simulink model "fft_biplex_test3"  (Simulink 7.6)
settings: Solver=ode45  StartTime=0.0  StopTime=5000  RelTol=1e-3
libraries: xbsIndex_r4 x1382, casper_library x82, monroe_library x27, xps_library x17, dspsigops x16, simulink x1
(part 1 of 13)
settings Model: Creator=monroe  LastModifiedBy=monroe

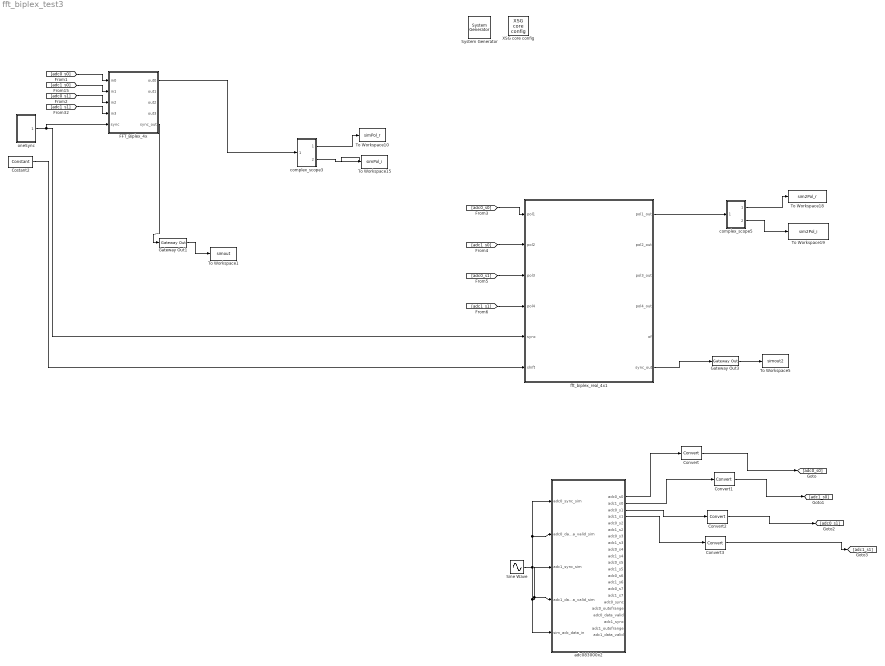
== system fft_biplex_test3 ==
  " System Generator" : xbsIndex_r4/ System Generator  Tag=genX  SystemSampleTime=-1  xilinxfamily=virtex5  part=xc5vsx95t  speed=-1  package=ff1136  synthesis_tool=XST  clock_wrapper=Clock Enables  directory=./spec_16in_extrabrams3/sysgen  testbench=off  simulink_period=1  sysclk_period=2.6667  dcm_input_clock_period=100  incr_netlist=off  trim_vbits=Everywhere in SubSystem  dbl_ovrd=According to Block Masks  core_generation=According to Block Masks  run_coregen=off  deprecated_control=off  eval_field=0  block_type=sysgen
      settings: block_version=11.4
  Convert{,1..3} (4 alike) : xbsIndex_r4/Convert  arith_type="Signed  (2's comp)"  n_bits=18  bin_pt=17  quantization=Truncate  overflow=Wrap  en=off  latency=0  dbl_ovrd=off  pipeline=off  block_type=convert
  Costant2 : xbsIndex_r4/Constant  arith_type=Signed (2's comp)  const=-1  n_bits=32  bin_pt=0  explicit_period=on  period=1  equ=P=C  opselect=C  inp2=PCIN>>17  opr=+  inp1=P  carry=CIN  dbl_ovrd=off  block_type=constant
      settings: block_version=11.4
  FFT_Biplex_4x : Subsystem  mask{FFTSize=10, coeff_bit_width=18*ones(1,8), input_bit_width=18, inter_stage_bit_width=18*ones(1,10), shift_arr=ones(1,10), max_distro_size_coeff=3, max_distro_size_delay=3, register_coeffs=0, stage_pre_delay=1, stage_mid_delay=1, stage_post_delay=0, bram_latency_fft=2, bram_latency_unscr=2, unscr_din_latency=0}
      mask prompts: FFTSize "FFT Size (2^?) points"; coeff_bit_width "Coefficient Bit Width"; input_bit_width "Input Bit Width"; inter_stage_bit_width "Inter-Stage Bit Widths"; shift_arr "Shift after n-th stage? (array of FFTSize elements, each a 0 or 1)"; max_distro_size_coeff "When to start putting Coefficients in BRAM (after 2^? elements)"; max_distro_size_delay "When to start putting Delays in BRAM (after 2^? latency)"; register_coeffs "Register Coefficients?"; stage_pre_delay "Stage Pre-delay? (0 or 1)"; stage_mid_delay "Stage Mid-Delay? (0 or 1)"; stage_post_delay "Stage Post-Delay? (0 or 1)"; bram_latency_fft "BRAM Latency (FFT)"; bram_latency_unscr "BRAM Latency (Unscrambler)"; unscr_din_latency "Unscrambler DIN Latency"
      mask init:
      | config.source=str2func('fft_biplex_4x_draw');
      | config.toplevel=gcb;
      | config.debug=0;
      | config.depend={'fft_biplex_4x_draw.m'};
      | xBlock(config,{FFTSize,coeff_bit_width,input_bit_width,inter_stage_bit_width,shift_arr,max_distro_size_coeff,max_distro_size_delay,register_coeffs,stage_pre_delay,stage_mid_delay,stage_post_delay,bram_latency_fft,bram_latency_unscr,unscr_din_latency});
  Gateway Out1 : xbsIndex_r4/Gateway Out  hdl_port=on  timing_constraint=None  locs_specified=off  LOCs={}  block_type=gatewayout
      settings: infoedit="Gateway out block.  Converts Xilinx fixed point inputs into ouputs of type Simulink integer, double, or fixed point.<br><br>Hardware notes:  In hardware these blocks become top level output ports or are discarded, depending on how they are configured."  block_version=11.4
  Gateway Out3 : xbsIndex_r4/Gateway Out  hdl_port=on  timing_constraint=None  locs_specified=off  LOCs={}  block_type=gatewayout
      settings: infoedit="Gateway out block.  Converts Xilinx fixed point inputs into ouputs of type Simulink integer, double, or fixed point.<br><br>Hardware notes:  In hardware these blocks become top level output ports or are discarded, depending on how they are configured."  block_version=11.4
  Sine Wave : Sin  Amplitude=.4  Frequency=1654.4/4096*pi*8  SampleTime=1/16
  To Workspace1 : ToWorkspace  VariableName=simout  SampleTime=-1  SaveFormat=Structure
  To Workspace10 : ToWorkspace  VariableName=simPol_r  SampleTime=-1  SaveFormat=Structure
  To Workspace15 : ToWorkspace  VariableName=simPol_i  SampleTime=-1  SaveFormat=Structure
  To Workspace18 : ToWorkspace  VariableName=sim2Pol_r  SampleTime=-1  SaveFormat=Structure
  To Workspace19 : ToWorkspace  VariableName=sim2Pol_i  SampleTime=-1  SaveFormat=Structure
  To Workspace5 : ToWorkspace  VariableName=simout2  SampleTime=-1  SaveFormat=Structure
  XSG core config : xps_library/XSG core config  Tag=xps:xsg  SystemSampleTime=-1  hw_sys=ROACH:sx95t  ibob_linux=off  clk_src=adc0_clk  iBOB_clk_src=sys_clk  BEE2_ctrl_clk_src=sys_clk  BEE2_usr_clk_src=sys_clk  ROACH_clk_src=adc0_clk  CORR_clk_src=sys_clk  gpio_clk_io_group=iBOB:sma  gpio_clk_bit_index=0  clk_rate=375  sample_period=1  synthesis_tool=XST  mpc_type=powerpc440_ext
  adc083000x2 : Subsystem  Tag=xps:adc083000x2  mask(adc_083000x2){use_adc0=on, use_adc1=on, demux_adc=off, clock_sync=off, verbose=on, using_ctrl=on, adc_clk_rate=1500, sample_period=1, bit_width=8}
      mask prompts: use_adc0 "Use ZD0K0?"; use_adc1 "Use ZDOK1?"; demux_adc "Demux ADCs by 2?"; clock_sync "Interleave 2 ADC boards?"; verbose "Verbose Block Creation?"; using_ctrl "Add ports for control registers?"; adc_clk_rate "ADC clock rate (MHz)"; sample_period "Sample Period"; bit_width "Output Bit Width"
      mask help:
      | The ADC block converts analog inputs to digital outputs.
      | Every clock cycle, the inputs are sampled and digitized to
      | 8 bit binary point numbers in the range of [-1, 1).
      |
      | Online block-specific documentation: http://casper.berkeley.edu/wiki/Adc083000
      mask Help: eval('xlWeb([getenv(''MLIB_ROOT''), ''\doc\html\sys_adc\sys_adc.html''])')
  complex_scope3 : Subsystem
  complex_scope5 : Subsystem
  fft_biplex_real_4x1 : Subsystem  AncestorBlock=casper_library/FFTs/fft_biplex_real_4x  mask(fft_biplex_real_4x){FFTSize=10, input_bit_width=8, coeff_bit_width=18, quantization=Truncate, overflow=Wrap, add_latency=2, mult_latency=3, bram_latency=3, arch=Virtex5, opt_target=Logic, coeffs_bit_limit=8, delays_bit_limit=9, specify_mult=off, mult_spec=, dsp48_adders=on, shifts=getfield( getfield( get_param( gcb,'UserData' ), 'parameters'),'shifts'), output_bit_widths=getfield( getfield( get_param( gcb,'UserData' ), 'parameters'),'output_bit_widths')}
      mask prompts: FFTSize "Size of FFT: (2^? pnts)"; input_bit_width "Input Bit Width"; coeff_bit_width "Coefficient Bit Width"; quantization "Quantization Behavior"; overflow "Overflow Behavior"; add_latency "Add Latency"; mult_latency "Mult Latency"; bram_latency "BRAM Latency"; arch "Architecture"; opt_target "Optimisation Target"; coeffs_bit_limit "Number bits above which to store stage's coefficients in BRAM (2^? bits)"; delays_bit_limit "Number bits above which to implement stage's delays in BRAM (2^? bits)"; specify_mult "Specify multiplier use (behavioral HDL if not specified)"; mult_spec "Multiplier specification (0=core, 1=embedded, 2=behavioural) (left=1st stage)"; dsp48_adders "Use DSP48s for adders"; shifts "Shift Schedule"; output_bit_widths "Output Bit Widths (vector len = nStages)"
      mask init:
      | fft_biplex_real_4x_init(gcb, ...
      |     'FFTSize', FFTSize, ...
      |     'input_bit_width', input_bit_width, ...
      |     'coeff_bit_width', coeff_bit_width, ...
      |     'quantization', quantization, ...
      |     'overflow', overflow, ...
      |     'add_latency', add_latency, ...
      |     'mult_latency', mult_latency, ...
      |     'bram_latency', bram_latency, ...
      |     'arch', arch, ...
      |     'opt_target', opt_target, ...
      |     'coeffs_bit_limit', coeffs_bit_limit, ...
      |     'delays_bit_limit', delays_bit_limit, ...    
      |     'specify_mult', specify_mult, ...
      |     'mult_spec', mult_spec, ...
      |     'dsp48_adders', dsp48_adders, ...
      |     'shifts', shifts, ...
      |     'output_bit_widths', output_bit_widths);
      settings: AttributesFormatString=FFTSize=10
      mask Help: eval('xlWeb(''http://casper.berkeley.edu/wiki/Fft_biplex_real_4x'')')
      mask StyleString: edit,edit,edit,popup(Truncate|Round  (unbiased: +/- Inf)|Round  (unbiased: Even Values)),popup(Wrap|Saturate|Error),edit,edit,edit,popup(Virtex2Pro|Virtex5),popup(Logic|Multipliers),edit,edit,checkbox,edit,checkbox,edit,edit
      mask CallbackString:
      | % fft_size = eval(get_param(gcb, 'FFTSize'));
      | % old_vec = eval(get_param(gcb, 'mult_spec'));
      | 
      | % vec = 2.*ones(1,fft_size);
      | % old_size = length(old_vec);
      | 
      | % if(old_size <= fft_size),
      | %     size = old_size;
      | % else,
      | %     size = fft_size;
      | % end
      | 
      | % for n = 1:size, vec(n) = old_vec(n); end
      | % set_param(gcb, 'mult_spec', mat2str(vec));||||||||||||specify_mult = get_param(gcb,'specify_mult');
      | visibs = get_param(gcb, 'MaskVisibilities');
      | enables = get_param(gcb, 'MaskEnables');
      | enables{14} = 'on';
      | if( strcmp(specify_mult,'off')), visibs{14} = 'off';
      | else, visibs{14} = 'on';
      | end
      | set_param(gcb, 'MaskVisibilities', visibs);
      | set_param(gcb, 'MaskEnables', enables);
      | |% vec = eval( get_param(gcb, 'mult_spec'));
      | % vec_size = length(vec);
      | % fft_size = eval( get_param(gcb, 'FFTSize'));
      | % new_vec = 2.*ones(1, fft_size);
      | 
      | % if(vec_size <= fft_size), size = vec_size;
      | % else size = fft_size;
      | % end
      | 
      | % for n=1:size
      | %    new_vec(n) = vec(n);
      | % end
      | % set_param(gcb, 'mult_spec', mat2str(new_vec));|||
  oneSync : Subsystem
  wires:
  [adc0_s0] -> FFT_Biplex_4x/1(in0)
  [adc1_s0] -> FFT_Biplex_4x/2(in1)
  [adc0_s1] -> FFT_Biplex_4x/3(in2)
  [adc1_s1] -> FFT_Biplex_4x/4(in3)
  oneSync/1(sync_out) -> fft_biplex_real_4x1/5(sync), FFT_Biplex_4x/5(sync)
  complex_scope3/1(Real) -> To Workspace10/1
  complex_scope3/2(Imag) -> To Workspace15/1
  FFT_Biplex_4x/5(sync_out) -> Gateway Out1/1
  Gateway Out1/1 -> To Workspace1/1
  [adc0_s0] -> fft_biplex_real_4x1/1(pol1)
  [adc1_s0] -> fft_biplex_real_4x1/2(pol2)
  [adc0_s1] -> fft_biplex_real_4x1/3(pol3)
  [adc1_s1] -> fft_biplex_real_4x1/4(pol4)
  complex_scope5/1(Real) -> To Workspace18/1
  complex_scope5/2(Imag) -> To Workspace19/1
  fft_biplex_real_4x1/1(pol1_out) -> complex_scope5/1(In1)
  Costant2/1 -> fft_biplex_real_4x1/6(shift)
  FFT_Biplex_4x/1(out0) -> complex_scope3/1(In1)
  Gateway Out3/1 -> To Workspace5/1
  fft_biplex_real_4x1/6(sync_out) -> Gateway Out3/1
  Sine Wave/1 -> adc083000x2/2(adc0_data_valid_sim), adc083000x2/1(adc0_sync_sim), adc083000x2/4(adc1_data_valid_sim), adc083000x2/3(adc1_sync_sim), adc083000x2/5(sim_adc_data_in)
  adc083000x2/1(adc0_s0) -> Convert/1
  adc083000x2/2(adc1_s0) -> Convert1/1
  adc083000x2/3(adc0_s1) -> Convert2/1
  adc083000x2/4(adc1_s1) -> Convert3/1
  Convert3/1 -> [adc1_s1]
  Convert2/1 -> [adc0_s1]
  Convert1/1 -> [adc1_s0]
  Convert/1 -> [adc0_s0]

== system fft_biplex_test3/FFT_Biplex_4x ==
  in0 : Inport
  in1 : Inport  Port=2
  in2 : Inport  Port=3
  in3 : Inport  Port=4
  sync : Inport  Port=5
  biplex_4x_unscr : Subsystem
  biplex_muxsel_gen : Subsystem
  coeff_slice10 : xbsIndex_r4/Slice  nbits=36  boolean_output=off  mode=Upper Bit Location + Width  bit1=-252  base1=MSB of Input  bit0=-252  base0=MSB of Input  dbl_ovrd=off  block_type=slice
  coeff_slice3 : xbsIndex_r4/Slice  nbits=36  boolean_output=off  mode=Upper Bit Location + Width  bit1=-0  base1=MSB of Input  bit0=-0  base0=MSB of Input  dbl_ovrd=off  block_type=slice
  coeff_slice4 : xbsIndex_r4/Slice  nbits=36  boolean_output=off  mode=Upper Bit Location + Width  bit1=-36  base1=MSB of Input  bit0=-36  base0=MSB of Input  dbl_ovrd=off  block_type=slice
  coeff_slice5 : xbsIndex_r4/Slice  nbits=36  boolean_output=off  mode=Upper Bit Location + Width  bit1=-72  base1=MSB of Input  bit0=-72  base0=MSB of Input  dbl_ovrd=off  block_type=slice
  coeff_slice6 : xbsIndex_r4/Slice  nbits=36  boolean_output=off  mode=Upper Bit Location + Width  bit1=-108  base1=MSB of Input  bit0=-108  base0=MSB of Input  dbl_ovrd=off  block_type=slice
  coeff_slice7 : xbsIndex_r4/Slice  nbits=36  boolean_output=off  mode=Upper Bit Location + Width  bit1=-144  base1=MSB of Input  bit0=-144  base0=MSB of Input  dbl_ovrd=off  block_type=slice
  coeff_slice8 : xbsIndex_r4/Slice  nbits=36  boolean_output=off  mode=Upper Bit Location + Width  bit1=-180  base1=MSB of Input  bit0=-180  base0=MSB of Input  dbl_ovrd=off  block_type=slice
  coeff_slice9 : xbsIndex_r4/Slice  nbits=36  boolean_output=off  mode=Upper Bit Location + Width  bit1=-216  base1=MSB of Input  bit0=-216  base0=MSB of Input  dbl_ovrd=off  block_type=slice
  cram0 : Subsystem
  cram1 : Subsystem
  sel_slice1 : xbsIndex_r4/Slice  nbits=1  boolean_output=on  mode=Upper Bit Location + Width  bit1=-0  base1=MSB of Input  bit0=-0  base0=MSB of Input  dbl_ovrd=off  block_type=slice
  sel_slice10 : xbsIndex_r4/Slice  nbits=1  boolean_output=on  mode=Upper Bit Location + Width  bit1=-9  base1=MSB of Input  bit0=-9  base0=MSB of Input  dbl_ovrd=off  block_type=slice
  sel_slice2 : xbsIndex_r4/Slice  nbits=1  boolean_output=on  mode=Upper Bit Location + Width  bit1=-1  base1=MSB of Input  bit0=-1  base0=MSB of Input  dbl_ovrd=off  block_type=slice
  sel_slice3 : xbsIndex_r4/Slice  nbits=1  boolean_output=on  mode=Upper Bit Location + Width  bit1=-2  base1=MSB of Input  bit0=-2  base0=MSB of Input  dbl_ovrd=off  block_type=slice
  sel_slice4 : xbsIndex_r4/Slice  nbits=1  boolean_output=on  mode=Upper Bit Location + Width  bit1=-3  base1=MSB of Input  bit0=-3  base0=MSB of Input  dbl_ovrd=off  block_type=slice
  sel_slice5 : xbsIndex_r4/Slice  nbits=1  boolean_output=on  mode=Upper Bit Location + Width  bit1=-4  base1=MSB of Input  bit0=-4  base0=MSB of Input  dbl_ovrd=off  block_type=slice
  sel_slice6 : xbsIndex_r4/Slice  nbits=1  boolean_output=on  mode=Upper Bit Location + Width  bit1=-5  base1=MSB of Input  bit0=-5  base0=MSB of Input  dbl_ovrd=off  block_type=slice
  sel_slice7 : xbsIndex_r4/Slice  nbits=1  boolean_output=on  mode=Upper Bit Location + Width  bit1=-6  base1=MSB of Input  bit0=-6  base0=MSB of Input  dbl_ovrd=off  block_type=slice
  sel_slice8 : xbsIndex_r4/Slice  nbits=1  boolean_output=on  mode=Upper Bit Location + Width  bit1=-7  base1=MSB of Input  bit0=-7  base0=MSB of Input  dbl_ovrd=off  block_type=slice
  sel_slice9 : xbsIndex_r4/Slice  nbits=1  boolean_output=on  mode=Upper Bit Location + Width  bit1=-8  base1=MSB of Input  bit0=-8  base0=MSB of Input  dbl_ovrd=off  block_type=slice
  stage_1 : Subsystem
  stage_10 : Subsystem
  stage_2 : Subsystem
  stage_3 : Subsystem
  stage_4 : Subsystem
  stage_5 : Subsystem
  stage_6 : Subsystem
  stage_7 : Subsystem
  stage_8 : Subsystem
  stage_9 : Subsystem
  out0 : Outport
  out1 : Outport  Port=2
  out2 : Outport  Port=3
  out3 : Outport  Port=4
  sync_out : Outport  Port=5
  wires:
  in0/1 -> cram0/1(in0)
  in1/1 -> cram0/2(in1)
  in2/1 -> cram1/1(in0)
  in3/1 -> cram1/2(in1)
  cram0/1(out) -> stage_1/1(a)
  cram1/1(out) -> stage_1/2(b)
  sel_slice1/1 -> stage_1/4(mux_sel)
  stage_1/1(a+bw) -> stage_2/1(a)
  stage_1/2(a-bw) -> stage_2/2(b)
  stage_1/3(sync_out) -> stage_2/3(sync)
  sel_slice2/1 -> stage_2/4(mux_sel)
  stage_2/1(a+bw) -> stage_3/1(a)
  stage_2/2(a-bw) -> stage_3/2(b)
  stage_2/3(sync_out) -> stage_3/3(sync)
  coeff_slice3/1 -> stage_3/4(coeff)
  sel_slice3/1 -> stage_3/5(mux_sel)
  stage_3/1(a+bw) -> stage_4/1(a)
  stage_3/2(a-bw) -> stage_4/2(b)
  stage_3/3(sync_out) -> stage_4/3(sync)
  coeff_slice4/1 -> stage_4/4(coeff)
  sel_slice4/1 -> stage_4/5(mux_sel)
  stage_4/1(a+bw) -> stage_5/1(a)
  stage_4/2(a-bw) -> stage_5/2(b)
  stage_4/3(sync_out) -> stage_5/3(sync)
  coeff_slice5/1 -> stage_5/4(coeff)
  sel_slice5/1 -> stage_5/5(mux_sel)
  stage_5/1(a+bw) -> stage_6/1(a)
  stage_5/2(a-bw) -> stage_6/2(b)
  stage_5/3(sync_out) -> stage_6/3(sync)
  coeff_slice6/1 -> stage_6/4(coeff)
  sel_slice6/1 -> stage_6/5(mux_sel)
  stage_6/1(a+bw) -> stage_7/1(a)
  stage_6/2(a-bw) -> stage_7/2(b)
  stage_6/3(sync_out) -> stage_7/3(sync)
  coeff_slice7/1 -> stage_7/4(coeff)
  sel_slice7/1 -> stage_7/5(mux_sel)
  stage_7/1(a+bw) -> stage_8/1(a)
  stage_7/2(a-bw) -> stage_8/2(b)
  stage_7/3(sync_out) -> stage_8/3(sync)
  coeff_slice8/1 -> stage_8/4(coeff)
  sel_slice8/1 -> stage_8/5(mux_sel)
  stage_8/1(a+bw) -> stage_9/1(a)
  stage_8/2(a-bw) -> stage_9/2(b)
  stage_8/3(sync_out) -> stage_9/3(sync)
  coeff_slice9/1 -> stage_9/4(coeff)
  sel_slice9/1 -> stage_9/5(mux_sel)
  stage_9/1(a+bw) -> stage_10/1(a)
  stage_9/2(a-bw) -> stage_10/2(b)
  stage_9/3(sync_out) -> stage_10/3(sync)
  coeff_slice10/1 -> stage_10/4(coeff)
  sel_slice10/1 -> stage_10/5(mux_sel)
  stage_10/1(a+bw) -> biplex_4x_unscr/1(even)
  stage_10/2(a-bw) -> biplex_4x_unscr/2(odd)
  biplex_muxsel_gen/3(sync_out) -> biplex_4x_unscr/3(sync)
  biplex_4x_unscr/1(pol1_out) -> out0/1
  biplex_4x_unscr/2(pol2_out) -> out1/1
  biplex_4x_unscr/3(pol3_out) -> out2/1
  biplex_4x_unscr/4(pol4_out) -> out3/1
  biplex_4x_unscr/5(sync_out) -> sync_out/1
  biplex_muxsel_gen/1(coeff) -> coeff_slice3/1, coeff_slice4/1, coeff_slice5/1, coeff_slice6/1, coeff_slice7/1, coeff_slice8/1, coeff_slice9/1, coeff_slice10/1
  biplex_muxsel_gen/2(sel) -> sel_slice1/1, sel_slice2/1, sel_slice3/1, sel_slice4/1, sel_slice5/1, sel_slice6/1, sel_slice7/1, sel_slice8/1, sel_slice9/1, sel_slice10/1
  sync/1 -> biplex_muxsel_gen/1(sync), stage_1/3(sync)

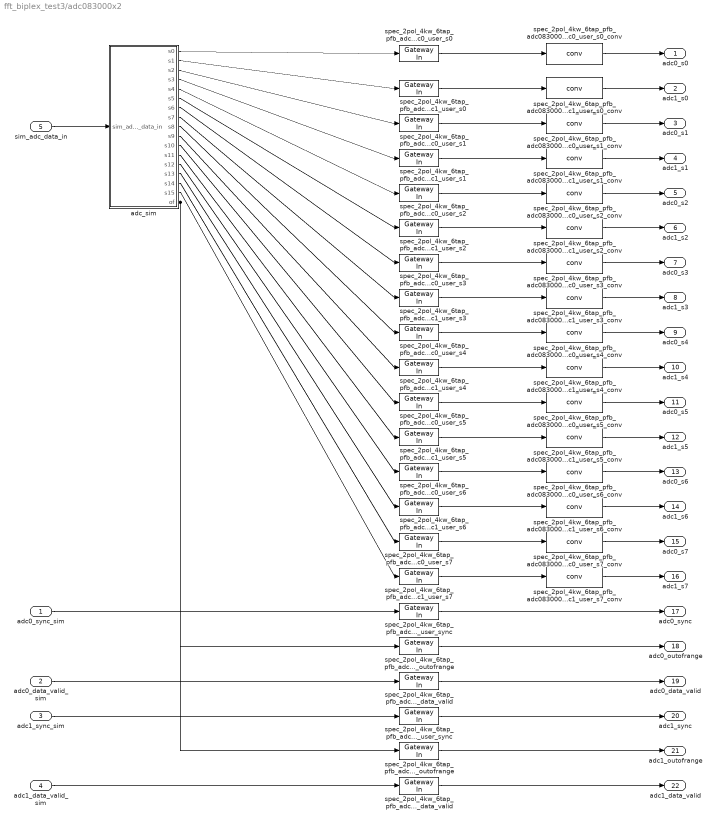
== system fft_biplex_test3/adc083000x2 ==
  adc0_sync_sim : Inport
  adc0_data_valid_sim : Inport  Port=2
  adc1_sync_sim : Inport  Port=3
  adc1_data_valid_sim : Inport  Port=4
  sim_adc_data_in : Inport  Port=5
  adc_sim : Subsystem  AncestorBlock=xps_library/ADCs/adc_sim  mask(adc_sim){nStreams=16, bit_width=8}
      mask prompts: nStreams "Number of Output Streams"; bit_width "Sample Bit Width"
      mask help:
      | This block simulates the behavior of a demuxed ADC, which takes
      | as input a waveform and returns digital samples in parallel at
      | a slower rate.
      |
      | This block is used to simulate the behavior
      mask init:
      | adc_sim_init(gcb, ...
      |     'nStreams', nStreams, ...
      |     'bit_width', bit_width);
  spec_2pol_4kw_6tap_pfb_adc083000x2_adc0_user_data_valid : xbsIndex_r4/Gateway In  arith_type=Unsigned  n_bits=1  bin_pt=0  quantization="Round  (unbiased: +/- Inf)"  overflow=Saturate  period=1  dbl_ovrd=off  timing_constraint=None  locs_specified=off  LOCs={}  hdl_port=on  block_type=gatewayin
      settings: infoedit="Gateway in block.  Converts inputs of type Simulink integer, double and fixed point to  Xilinx fixed point type.<br><br>Hardware notes:  In hardware these blocks become top level input ports."
  spec_2pol_4kw_6tap_pfb_adc083000x2_adc0_user_outofrange : xbsIndex_r4/Gateway In  arith_type=Unsigned  n_bits=4  bin_pt=0  quantization="Round  (unbiased: +/- Inf)"  overflow=Saturate  period=1  dbl_ovrd=off  timing_constraint=None  locs_specified=off  LOCs={}  hdl_port=on  block_type=gatewayin
      settings: infoedit="Gateway in block.  Converts inputs of type Simulink integer, double and fixed point to  Xilinx fixed point type.<br><br>Hardware notes:  In hardware these blocks become top level input ports."
  spec_2pol_4kw_6tap_pfb_adc083000x2_adc0_user_s{0..7} (8 alike) : xbsIndex_r4/Gateway In  arith_type=Unsigned  n_bits=8  bin_pt=0  quantization="Round  (unbiased: +/- Inf)"  overflow=Saturate  period=1  dbl_ovrd=off  timing_constraint=None  locs_specified=off  LOCs={}  hdl_port=on  block_type=gatewayin
      settings: infoedit="Gateway in block.  Converts inputs of type Simulink integer, double and fixed point to  Xilinx fixed point type.<br><br>Hardware notes:  In hardware these blocks become top level input ports."
  spec_2pol_4kw_6tap_pfb_adc083000x2_adc0_user_s0_conv : xps_library/ADCs/conv  SystemSampleTime=-1  bit_width=8
  spec_2pol_4kw_6tap_pfb_adc083000x2_adc0_user_s1_conv : xps_library/ADCs/conv  SystemSampleTime=-1  bit_width=8
  spec_2pol_4kw_6tap_pfb_adc083000x2_adc0_user_s2_conv : xps_library/ADCs/conv  SystemSampleTime=-1  bit_width=8
  spec_2pol_4kw_6tap_pfb_adc083000x2_adc0_user_s3_conv : xps_library/ADCs/conv  SystemSampleTime=-1  bit_width=8
  spec_2pol_4kw_6tap_pfb_adc083000x2_adc0_user_s4_conv : xps_library/ADCs/conv  SystemSampleTime=-1  bit_width=8
  spec_2pol_4kw_6tap_pfb_adc083000x2_adc0_user_s5_conv : xps_library/ADCs/conv  SystemSampleTime=-1  bit_width=8
  spec_2pol_4kw_6tap_pfb_adc083000x2_adc0_user_s6_conv : xps_library/ADCs/conv  SystemSampleTime=-1  bit_width=8
  spec_2pol_4kw_6tap_pfb_adc083000x2_adc0_user_s7_conv : xps_library/ADCs/conv  SystemSampleTime=-1  bit_width=8
  spec_2pol_4kw_6tap_pfb_adc083000x2_adc0_user_sync : xbsIndex_r4/Gateway In  arith_type=Unsigned  n_bits=4  bin_pt=0  quantization="Round  (unbiased: +/- Inf)"  overflow=Saturate  period=1  dbl_ovrd=off  timing_constraint=None  locs_specified=off  LOCs={}  hdl_port=on  block_type=gatewayin
      settings: infoedit="Gateway in block.  Converts inputs of type Simulink integer, double and fixed point to  Xilinx fixed point type.<br><br>Hardware notes:  In hardware these blocks become top level input ports."
  spec_2pol_4kw_6tap_pfb_adc083000x2_adc1_user_data_valid : xbsIndex_r4/Gateway In  arith_type=Unsigned  n_bits=1  bin_pt=0  quantization="Round  (unbiased: +/- Inf)"  overflow=Saturate  period=1  dbl_ovrd=off  timing_constraint=None  locs_specified=off  LOCs={}  hdl_port=on  block_type=gatewayin
      settings: infoedit="Gateway in block.  Converts inputs of type Simulink integer, double and fixed point to  Xilinx fixed point type.<br><br>Hardware notes:  In hardware these blocks become top level input ports."
  spec_2pol_4kw_6tap_pfb_adc083000x2_adc1_user_outofrange : xbsIndex_r4/Gateway In  arith_type=Unsigned  n_bits=4  bin_pt=0  quantization="Round  (unbiased: +/- Inf)"  overflow=Saturate  period=1  dbl_ovrd=off  timing_constraint=None  locs_specified=off  LOCs={}  hdl_port=on  block_type=gatewayin
      settings: infoedit="Gateway in block.  Converts inputs of type Simulink integer, double and fixed point to  Xilinx fixed point type.<br><br>Hardware notes:  In hardware these blocks become top level input ports."
  spec_2pol_4kw_6tap_pfb_adc083000x2_adc1_user_s{0..7} (8 alike) : xbsIndex_r4/Gateway In  arith_type=Unsigned  n_bits=8  bin_pt=0  quantization="Round  (unbiased: +/- Inf)"  overflow=Saturate  period=1  dbl_ovrd=off  timing_constraint=None  locs_specified=off  LOCs={}  hdl_port=on  block_type=gatewayin
      settings: infoedit="Gateway in block.  Converts inputs of type Simulink integer, double and fixed point to  Xilinx fixed point type.<br><br>Hardware notes:  In hardware these blocks become top level input ports."
  spec_2pol_4kw_6tap_pfb_adc083000x2_adc1_user_s0_conv : xps_library/ADCs/conv  SystemSampleTime=-1  bit_width=8
  spec_2pol_4kw_6tap_pfb_adc083000x2_adc1_user_s1_conv : xps_library/ADCs/conv  SystemSampleTime=-1  bit_width=8
  spec_2pol_4kw_6tap_pfb_adc083000x2_adc1_user_s2_conv : xps_library/ADCs/conv  SystemSampleTime=-1  bit_width=8
  spec_2pol_4kw_6tap_pfb_adc083000x2_adc1_user_s3_conv : xps_library/ADCs/conv  SystemSampleTime=-1  bit_width=8
  spec_2pol_4kw_6tap_pfb_adc083000x2_adc1_user_s4_conv : xps_library/ADCs/conv  SystemSampleTime=-1  bit_width=8
  spec_2pol_4kw_6tap_pfb_adc083000x2_adc1_user_s5_conv : xps_library/ADCs/conv  SystemSampleTime=-1  bit_width=8
  spec_2pol_4kw_6tap_pfb_adc083000x2_adc1_user_s6_conv : xps_library/ADCs/conv  SystemSampleTime=-1  bit_width=8
  spec_2pol_4kw_6tap_pfb_adc083000x2_adc1_user_s7_conv : xps_library/ADCs/conv  SystemSampleTime=-1  bit_width=8
  spec_2pol_4kw_6tap_pfb_adc083000x2_adc1_user_sync : xbsIndex_r4/Gateway In  arith_type=Unsigned  n_bits=4  bin_pt=0  quantization="Round  (unbiased: +/- Inf)"  overflow=Saturate  period=1  dbl_ovrd=off  timing_constraint=None  locs_specified=off  LOCs={}  hdl_port=on  block_type=gatewayin
      settings: infoedit="Gateway in block.  Converts inputs of type Simulink integer, double and fixed point to  Xilinx fixed point type.<br><br>Hardware notes:  In hardware these blocks become top level input ports."
  adc0_s0 : Outport
  adc1_s0 : Outport  Port=2
  adc0_s1 : Outport  Port=3
  adc1_s1 : Outport  Port=4
  adc0_s2 : Outport  Port=5
  adc1_s2 : Outport  Port=6
  adc0_s3 : Outport  Port=7
  adc1_s3 : Outport  Port=8
  adc0_s4 : Outport  Port=9
  adc1_s4 : Outport  Port=10
  adc0_s5 : Outport  Port=11
  adc1_s5 : Outport  Port=12
  adc0_s6 : Outport  Port=13
  adc1_s6 : Outport  Port=14
  adc0_s7 : Outport  Port=15
  adc1_s7 : Outport  Port=16
  adc0_sync : Outport  Port=17
  adc0_outofrange : Outport  Port=18
  adc0_data_valid : Outport  Port=19
  adc1_sync : Outport  Port=20
  adc1_outofrange : Outport  Port=21
  adc1_data_valid : Outport  Port=22
  wires:
  spec_2pol_4kw_6tap_pfb_adc083000x2_adc1_user_data_valid/1 -> adc1_data_valid/1
  adc1_data_valid_sim/1 -> spec_2pol_4kw_6tap_pfb_adc083000x2_adc1_user_data_valid/1
  spec_2pol_4kw_6tap_pfb_adc083000x2_adc1_user_outofrange/1 -> adc1_outofrange/1
  spec_2pol_4kw_6tap_pfb_adc083000x2_adc1_user_sync/1 -> adc1_sync/1
  adc1_sync_sim/1 -> spec_2pol_4kw_6tap_pfb_adc083000x2_adc1_user_sync/1
  spec_2pol_4kw_6tap_pfb_adc083000x2_adc0_user_data_valid/1 -> adc0_data_valid/1
  adc0_data_valid_sim/1 -> spec_2pol_4kw_6tap_pfb_adc083000x2_adc0_user_data_valid/1
  spec_2pol_4kw_6tap_pfb_adc083000x2_adc0_user_outofrange/1 -> adc0_outofrange/1
  adc_sim/17(of) -> spec_2pol_4kw_6tap_pfb_adc083000x2_adc1_user_outofrange/1, spec_2pol_4kw_6tap_pfb_adc083000x2_adc0_user_outofrange/1
  spec_2pol_4kw_6tap_pfb_adc083000x2_adc0_user_sync/1 -> adc0_sync/1
  adc0_sync_sim/1 -> spec_2pol_4kw_6tap_pfb_adc083000x2_adc0_user_sync/1
  spec_2pol_4kw_6tap_pfb_adc083000x2_adc1_user_s7_conv/1 -> adc1_s7/1
  spec_2pol_4kw_6tap_pfb_adc083000x2_adc1_user_s7/1 -> spec_2pol_4kw_6tap_pfb_adc083000x2_adc1_user_s7_conv/1
  adc_sim/16(s15) -> spec_2pol_4kw_6tap_pfb_adc083000x2_adc1_user_s7/1
  spec_2pol_4kw_6tap_pfb_adc083000x2_adc0_user_s7_conv/1 -> adc0_s7/1
  spec_2pol_4kw_6tap_pfb_adc083000x2_adc0_user_s7/1 -> spec_2pol_4kw_6tap_pfb_adc083000x2_adc0_user_s7_conv/1
  adc_sim/15(s14) -> spec_2pol_4kw_6tap_pfb_adc083000x2_adc0_user_s7/1
  spec_2pol_4kw_6tap_pfb_adc083000x2_adc1_user_s6_conv/1 -> adc1_s6/1
  spec_2pol_4kw_6tap_pfb_adc083000x2_adc1_user_s6/1 -> spec_2pol_4kw_6tap_pfb_adc083000x2_adc1_user_s6_conv/1
  adc_sim/14(s13) -> spec_2pol_4kw_6tap_pfb_adc083000x2_adc1_user_s6/1
  spec_2pol_4kw_6tap_pfb_adc083000x2_adc0_user_s6_conv/1 -> adc0_s6/1
  spec_2pol_4kw_6tap_pfb_adc083000x2_adc0_user_s6/1 -> spec_2pol_4kw_6tap_pfb_adc083000x2_adc0_user_s6_conv/1
  adc_sim/13(s12) -> spec_2pol_4kw_6tap_pfb_adc083000x2_adc0_user_s6/1
  spec_2pol_4kw_6tap_pfb_adc083000x2_adc1_user_s5_conv/1 -> adc1_s5/1
  spec_2pol_4kw_6tap_pfb_adc083000x2_adc1_user_s5/1 -> spec_2pol_4kw_6tap_pfb_adc083000x2_adc1_user_s5_conv/1
  adc_sim/12(s11) -> spec_2pol_4kw_6tap_pfb_adc083000x2_adc1_user_s5/1
  spec_2pol_4kw_6tap_pfb_adc083000x2_adc0_user_s5_conv/1 -> adc0_s5/1
  spec_2pol_4kw_6tap_pfb_adc083000x2_adc0_user_s5/1 -> spec_2pol_4kw_6tap_pfb_adc083000x2_adc0_user_s5_conv/1
  adc_sim/11(s10) -> spec_2pol_4kw_6tap_pfb_adc083000x2_adc0_user_s5/1
  spec_2pol_4kw_6tap_pfb_adc083000x2_adc1_user_s4_conv/1 -> adc1_s4/1
  spec_2pol_4kw_6tap_pfb_adc083000x2_adc1_user_s4/1 -> spec_2pol_4kw_6tap_pfb_adc083000x2_adc1_user_s4_conv/1
  adc_sim/10(s9) -> spec_2pol_4kw_6tap_pfb_adc083000x2_adc1_user_s4/1
  spec_2pol_4kw_6tap_pfb_adc083000x2_adc0_user_s4_conv/1 -> adc0_s4/1
  spec_2pol_4kw_6tap_pfb_adc083000x2_adc0_user_s4/1 -> spec_2pol_4kw_6tap_pfb_adc083000x2_adc0_user_s4_conv/1
  adc_sim/9(s8) -> spec_2pol_4kw_6tap_pfb_adc083000x2_adc0_user_s4/1
  spec_2pol_4kw_6tap_pfb_adc083000x2_adc1_user_s3_conv/1 -> adc1_s3/1
  spec_2pol_4kw_6tap_pfb_adc083000x2_adc1_user_s3/1 -> spec_2pol_4kw_6tap_pfb_adc083000x2_adc1_user_s3_conv/1
  adc_sim/8(s7) -> spec_2pol_4kw_6tap_pfb_adc083000x2_adc1_user_s3/1
  spec_2pol_4kw_6tap_pfb_adc083000x2_adc0_user_s3_conv/1 -> adc0_s3/1
  spec_2pol_4kw_6tap_pfb_adc083000x2_adc0_user_s3/1 -> spec_2pol_4kw_6tap_pfb_adc083000x2_adc0_user_s3_conv/1
  adc_sim/7(s6) -> spec_2pol_4kw_6tap_pfb_adc083000x2_adc0_user_s3/1
  spec_2pol_4kw_6tap_pfb_adc083000x2_adc1_user_s2_conv/1 -> adc1_s2/1
  spec_2pol_4kw_6tap_pfb_adc083000x2_adc1_user_s2/1 -> spec_2pol_4kw_6tap_pfb_adc083000x2_adc1_user_s2_conv/1
  adc_sim/6(s5) -> spec_2pol_4kw_6tap_pfb_adc083000x2_adc1_user_s2/1
  spec_2pol_4kw_6tap_pfb_adc083000x2_adc0_user_s2_conv/1 -> adc0_s2/1
  spec_2pol_4kw_6tap_pfb_adc083000x2_adc0_user_s2/1 -> spec_2pol_4kw_6tap_pfb_adc083000x2_adc0_user_s2_conv/1
  adc_sim/5(s4) -> spec_2pol_4kw_6tap_pfb_adc083000x2_adc0_user_s2/1
  spec_2pol_4kw_6tap_pfb_adc083000x2_adc1_user_s1_conv/1 -> adc1_s1/1
  spec_2pol_4kw_6tap_pfb_adc083000x2_adc1_user_s1/1 -> spec_2pol_4kw_6tap_pfb_adc083000x2_adc1_user_s1_conv/1
  adc_sim/4(s3) -> spec_2pol_4kw_6tap_pfb_adc083000x2_adc1_user_s1/1
  spec_2pol_4kw_6tap_pfb_adc083000x2_adc0_user_s1_conv/1 -> adc0_s1/1
  spec_2pol_4kw_6tap_pfb_adc083000x2_adc0_user_s1/1 -> spec_2pol_4kw_6tap_pfb_adc083000x2_adc0_user_s1_conv/1
  adc_sim/3(s2) -> spec_2pol_4kw_6tap_pfb_adc083000x2_adc0_user_s1/1
  spec_2pol_4kw_6tap_pfb_adc083000x2_adc1_user_s0_conv/1 -> adc1_s0/1
  spec_2pol_4kw_6tap_pfb_adc083000x2_adc1_user_s0/1 -> spec_2pol_4kw_6tap_pfb_adc083000x2_adc1_user_s0_conv/1
  adc_sim/2(s1) -> spec_2pol_4kw_6tap_pfb_adc083000x2_adc1_user_s0/1
  spec_2pol_4kw_6tap_pfb_adc083000x2_adc0_user_s0_conv/1 -> adc0_s0/1
  spec_2pol_4kw_6tap_pfb_adc083000x2_adc0_user_s0/1 -> spec_2pol_4kw_6tap_pfb_adc083000x2_adc0_user_s0_conv/1
  adc_sim/1(s0) -> spec_2pol_4kw_6tap_pfb_adc083000x2_adc0_user_s0/1
  sim_adc_data_in/1 -> adc_sim/1(sim_adc_data_in)

== system fft_biplex_test3/complex_scope3 ==
  In1 : Inport
  Gateway Out15 : xbsIndex_r4/Gateway Out  hdl_port=on  timing_constraint=None  locs_specified=off  LOCs={}  block_type=gatewayout
      settings: infoedit="Gateway out block.  Converts Xilinx fixed point inputs into ouputs of type Simulink integer, double, or fixed point.<br><br>Hardware notes:  In hardware these blocks become top level output ports or are discarded, depending on how they are configured."  block_version=11.4
  Gateway Out16 : xbsIndex_r4/Gateway Out  hdl_port=on  timing_constraint=None  locs_specified=off  LOCs={}  block_type=gatewayout
      settings: infoedit="Gateway out block.  Converts Xilinx fixed point inputs into ouputs of type Simulink integer, double, or fixed point.<br><br>Hardware notes:  In hardware these blocks become top level output ports or are discarded, depending on how they are configured."  block_version=11.4
  Reinterpret : xbsIndex_r4/Reinterpret  force_arith_type=on  arith_type="Signed  (2's comp)"  force_bin_pt=on  bin_pt=17  block_type=reinterpret
      settings: infoedit="Changes signal type without altering the binary representation.   You can changed the signal between signed and unsigned, and relocate the binary point.<br><br>Hardware notes: In hardware this block costs nothing.<br><br>Example:  Suppose the input is 6 bits wide, signed, with 2 fractional bits, and the output is forced to unsigned with 0 fractional bits.  Then an input of -2.0 (1110.00 in binary 2's complement) becomes an output of 56 (111000 in binary)."
  Reinterpret1 : xbsIndex_r4/Reinterpret  force_arith_type=on  arith_type="Signed  (2's comp)"  force_bin_pt=on  bin_pt=17  block_type=reinterpret
      settings: infoedit="Changes signal type without altering the binary representation.   You can changed the signal between signed and unsigned, and relocate the binary point.<br><br>Hardware notes: In hardware this block costs nothing.<br><br>Example:  Suppose the input is 6 bits wide, signed, with 2 fractional bits, and the output is forced to unsigned with 0 fractional bits.  Then an input of -2.0 (1110.00 in binary 2's complement) becomes an output of 56 (111000 in binary)."
  c_to_ri : casper_library/Misc/c_to_ri  SystemSampleTime=-1  n_bits=18  bin_pt=17
      settings: AttributesFormatString=18_17 r/i
  Real : Outport
  Imag : Outport  Port=2
  wires:
  c_to_ri/1 -> Reinterpret/1
  c_to_ri/2 -> Reinterpret1/1
  Reinterpret/1 -> Gateway Out15/1
  Reinterpret1/1 -> Gateway Out16/1
  Gateway Out15/1 -> Real/1
  In1/1 -> c_to_ri/1
  Gateway Out16/1 -> Imag/1

== system fft_biplex_test3/complex_scope5 ==
  In1 : Inport
  Gateway Out15 : xbsIndex_r4/Gateway Out  hdl_port=on  timing_constraint=None  locs_specified=off  LOCs={}  block_type=gatewayout
      settings: infoedit="Gateway out block.  Converts Xilinx fixed point inputs into ouputs of type Simulink integer, double, or fixed point.<br><br>Hardware notes:  In hardware these blocks become top level output ports or are discarded, depending on how they are configured."  block_version=11.4
  Gateway Out16 : xbsIndex_r4/Gateway Out  hdl_port=on  timing_constraint=None  locs_specified=off  LOCs={}  block_type=gatewayout
      settings: infoedit="Gateway out block.  Converts Xilinx fixed point inputs into ouputs of type Simulink integer, double, or fixed point.<br><br>Hardware notes:  In hardware these blocks become top level output ports or are discarded, depending on how they are configured."  block_version=11.4
  Reinterpret : xbsIndex_r4/Reinterpret  force_arith_type=on  arith_type="Signed  (2's comp)"  force_bin_pt=on  bin_pt=17  block_type=reinterpret
      settings: infoedit="Changes signal type without altering the binary representation.   You can changed the signal between signed and unsigned, and relocate the binary point.<br><br>Hardware notes: In hardware this block costs nothing.<br><br>Example:  Suppose the input is 6 bits wide, signed, with 2 fractional bits, and the output is forced to unsigned with 0 fractional bits.  Then an input of -2.0 (1110.00 in binary 2's complement) becomes an output of 56 (111000 in binary)."
  Reinterpret1 : xbsIndex_r4/Reinterpret  force_arith_type=on  arith_type="Signed  (2's comp)"  force_bin_pt=on  bin_pt=17  block_type=reinterpret
      settings: infoedit="Changes signal type without altering the binary representation.   You can changed the signal between signed and unsigned, and relocate the binary point.<br><br>Hardware notes: In hardware this block costs nothing.<br><br>Example:  Suppose the input is 6 bits wide, signed, with 2 fractional bits, and the output is forced to unsigned with 0 fractional bits.  Then an input of -2.0 (1110.00 in binary 2's complement) becomes an output of 56 (111000 in binary)."
  c_to_ri : casper_library/Misc/c_to_ri  SystemSampleTime=-1  n_bits=18  bin_pt=17
      settings: AttributesFormatString=18_17 r/i
  Real : Outport
  Imag : Outport  Port=2
  wires:
  Gateway Out16/1 -> Imag/1
  In1/1 -> c_to_ri/1
  Gateway Out15/1 -> Real/1
  Reinterpret1/1 -> Gateway Out16/1
  Reinterpret/1 -> Gateway Out15/1
  c_to_ri/2 -> Reinterpret1/1
  c_to_ri/1 -> Reinterpret/1

== system fft_biplex_test3/fft_biplex_real_4x1 ==
  pol1 : Inport
  pol2 : Inport  Port=2
  pol3 : Inport  Port=3
  pol4 : Inport  Port=4
  sync : Inport  Port=5
  shift : Inport  Port=6
  bi_real_unscr_4x : Subsystem  mask{FFTSize=5, bram_latency=3, input_bit_width=18}
      mask prompts: FFTSize "Size of FFT (2^?):"; bram_latency "BRAM Latency"; input_bit_width "Input Bit Width"
      mask init:
      | blk = gcb;
      | if same_state(blk, 'FFTSize', FFTSize, 'bram_latency', bram_latency), return, end
      | set_param([blk,'/reorder'],'map', mat2str(bit_reverse(0:2^(FFTSize-1)-1, FFTSize-1)));
      | set_param([blk,'/reorder'],'bram_latency', num2str(bram_latency));
      | set_param([blk,'/reorder1'],'map', mat2str(bit_reverse(2^(FFTSize-1)-1:-1:0, FFTSize-1)));
      | set_param([blk,'/reorder1'],'bram_latency', num2str(bram_latency));
      | set_param([blk,'/reorder2'],'map', mat2str(2^(FFTSize-1)-1:-1:0));
      | set_param([blk,'/reorder2'],'bram_latency', num2str(bram_latency));
      | save_state(blk, 'FFTSize', FFTSize, 'bram_latency', bram_latency);
  biplex_core : Subsystem  mask(biplex_core){FFTSize=10, input_bit_width=8, coeff_bit_width=18, quantization=Truncate, overflow=Wrap, add_latency=2, mult_latency=3, bram_latency=3, arch=Virtex5, opt_target=Logic, coeffs_bit_limit=8, delays_bit_limit=9, specify_mult=off, mult_spec=, dsp48_adders=on, shifts=[1                                      1                                      1                                      1                                      1                                      1                                      1                                      1                                      1                                      1], output_bit_widths=[18                                     18                                     18                                     18                                     18                                     18                                     18                                     18                                     18                                     18]}
      mask prompts: FFTSize "Size of FFT: (2^? pnts)"; input_bit_width "Input/Output Bit Width"; coeff_bit_width "Coefficient Bit Width"; quantization "Quantization Behavior"; overflow "Overflow Behavior"; add_latency "Add Latency"; mult_latency "Mult Latency"; bram_latency "BRAM Latency"; arch "Architecture"; opt_target "Optimisation Target"; coeffs_bit_limit "Number bits above which to store stage's coefficients in BRAM (2^? bits)"; delays_bit_limit "Number bits above which to implent stage's delays in BRAM (2^? bits)"; specify_mult "Specify multiplier use (behavioural HDL if not specified)"; mult_spec "Multiplier specification (0=core, 1=embedded, 2=behavioural) (left=1st stage)"; dsp48_adders "Use DSP48s for adders"; shifts "Shift Schedule"; output_bit_widths "Output Bit Width Vector (len = nStages)"
      mask init:
      | biplex_core_init(gcb,...
      |     'FFTSize', FFTSize,...
      |     'input_bit_width', input_bit_width,...
      |     'coeff_bit_width', coeff_bit_width,...
      |     'quantization', quantization,...
      |     'overflow', overflow,...
      |     'add_latency', add_latency,...
      |     'mult_latency', mult_latency,...
      |     'bram_latency', bram_latency,...
      |     'arch', arch, ...
      |     'opt_target', opt_target, ...
      |     'coeffs_bit_limit', coeffs_bit_limit, ...
      |     'delays_bit_limit', delays_bit_limit, ...
      |     'specify_mult', specify_mult, ...
      |     'mult_spec', mult_spec, ...
      |     'dsp48_adders', dsp48_adders, ...
      |     'shifts', shifts, ...
      |     'output_bit_widths', output_bit_widths);
      settings: AttributesFormatString=|
      | FFTSize=10,
      |  opt_target=Logic,
      |  arch=Virtex5
      mask StyleString: edit,edit,edit,popup(Truncate|Round  (unbiased: +/- Inf)|Round  (unbiased: Even Values)),popup(Wrap|Saturate|Error),edit,edit,edit,popup(Virtex2Pro|Virtex5),popup(Logic|Multipliers),edit,edit,checkbox,edit,checkbox,edit,edit
      mask CallbackString:
      | % fft_size = eval(get_param(gcb, 'FFTSize'));
      | % old_vec = eval(get_param(gcb, 'mult_spec'));
      | 
      | % vec = 2.*ones(1,fft_size);
      | % old_size = length(old_vec);
      | 
      | % if(old_size <= fft_size),
      | %    size = old_size;
      | % else,
      | %     size = fft_size;
      | % end
      | 
      | % for n = 1:size, vec(n) = old_vec(n); end
      | % set_param(gcb, 'mult_spec', mat2str(vec));||||||||||||specify_mult = get_param(gcb,'specify_mult');
      | visibs = get_param(gcb,'MaskVisibilities');
      | if( strcmp(specify_mult,'off')), visibs{14} = 'off';
      | else, visibs{14} = 'on';
      | end
      | set_param(gcb, 'MaskVisibilities', visibs);
      | enables = get_param(gcb,'MaskVisibilities');
      | enables{14} = 'on';
      | set_param(gcb, 'MaskEnables', enables);
      | |% vec = eval( get_param(gcb, 'mult_spec'));
      | % vec_size = length(vec);
      | % fft_size = eval( get_param(gcb, 'FFTSize'));
      | % new_vec = 2.*ones(1, fft_size);
      | 
      | % if(vec_size <= fft_size), size = vec_size;
      | % else size = fft_size;
      | % end
      | 
      | % for n=1:size
      | %     new_vec(n) = vec(n);
      | % end
      | % set_param(gcb, 'mult_spec', mat2str(new_vec));|||
  ri_to_c : Subsystem
  ri_to_c1 : Subsystem
  pol1_out : Outport
  pol2_out : Outport  Port=2
  pol3_out : Outport  Port=3
  pol4_out : Outport  Port=4
  of : Outport  Port=5
  sync_out : Outport  Port=6
  wires:
  biplex_core/4(sync_out) -> bi_real_unscr_4x/3(sync)
  biplex_core/2(out2) -> bi_real_unscr_4x/2(odd)
  biplex_core/1(out1) -> bi_real_unscr_4x/1(even)
  biplex_core/3(of) -> of/1
  pol1/1 -> ri_to_c/1(re)
  ri_to_c/1(c) -> biplex_core/1(pol1)
  pol2/1 -> ri_to_c/2(im)
  pol3/1 -> ri_to_c1/1(re)
  ri_to_c1/1(c) -> biplex_core/2(pol2)
  pol4/1 -> ri_to_c1/2(im)
  sync/1 -> biplex_core/3(sync)
  shift/1 -> biplex_core/4(shift)
  bi_real_unscr_4x/1(pol1_out) -> pol1_out/1
  bi_real_unscr_4x/2(pol2_out) -> pol2_out/1
  bi_real_unscr_4x/3(pol3_out) -> pol3_out/1
  bi_real_unscr_4x/4(pol4_out) -> pol4_out/1
  bi_real_unscr_4x/5(sync_out) -> sync_out/1

== system fft_biplex_test3/oneSync ==
  Costant3 : xbsIndex_r4/Constant  arith_type=Unsigned  const=2^11 -1  n_bits=11  bin_pt=0  explicit_period=on  period=1  equ=P=C  opselect=C  inp2=PCIN>>17  opr=+  inp1=P  carry=CIN  dbl_ovrd=off  block_type=constant
      settings: block_version=11.4
  Counter1 : xbsIndex_r4/Counter  cnt_type=Free Running  cnt_to=2^11-2  operation=Up  start_count=0  cnt_by_val=1  arith_type=Unsigned  n_bits=11  bin_pt=0  load_pin=off  rst=off  en=off  explicit_period=on  period=1  dbl_ovrd=off  use_behavioral_HDL=off  implementation=Fabric  block_type=counter
      settings: block_version=11.3
  Inverter : xbsIndex_r4/Inverter  en=off  latency=0  dbl_ovrd=off  block_type=inv
      settings: block_version=11.4
  Logical : xbsIndex_r4/Logical  logical_function=OR  inputs=2  en=off  latency=0  precision=Full  arith_type=Unsigned  n_bits=16  bin_pt=0  align_bp=on  dbl_ovrd=off  block_type=logical
      settings: block_version=11.4
  Logical1 : xbsIndex_r4/Logical  logical_function=AND  inputs=2  en=off  latency=2  precision=Full  arith_type=Unsigned  n_bits=16  bin_pt=0  align_bp=on  dbl_ovrd=off  block_type=logical
      settings: block_version=11.4
  Relational1 : xbsIndex_r4/Relational  mode=a=b  en=off  latency=1  dbl_ovrd=off  block_type=relational
  hadSync : xbsIndex_r4/Register  init=0  rst=off  en=off  dbl_ovrd=off  block_type=register
      settings: block_version=11.4
  sync_out : Outport
  wires:
  hadSync/1 -> Logical/2, Inverter/1
  Logical/1 -> hadSync/1
  Logical1/1 -> sync_out/1, Logical/1
  Relational1/1 -> Logical1/2
  Inverter/1 -> Logical1/1
  Costant3/1 -> Relational1/2
  Counter1/1 -> Relational1/1

== system fft_biplex_test3/FFT_Biplex_4x/biplex_4x_unscr ==
  even : Inport
  odd : Inport  Port=2
  sync : Inport  Port=3
  Constant1 : xbsIndex_r4/Constant  arith_type=Unsigned  const=511  n_bits=10  bin_pt=0  explicit_period=on  period=1  equ=P=C  opselect=C  inp2=PCIN>>17  opr=+  inp1=P  carry=CIN  dbl_ovrd=off  block_type=constant
  Constant2 : xbsIndex_r4/Constant  arith_type=Unsigned  const=1023  n_bits=10  bin_pt=0  explicit_period=on  period=1  equ=P=C  opselect=C  inp2=PCIN>>17  opr=+  inp1=P  carry=CIN  dbl_ovrd=off  block_type=constant
  Counter : xbsIndex_r4/Counter  cnt_type=Free Running  cnt_to=Inf  operation=Up  start_count=0  cnt_by_val=1  arith_type=Unsigned  n_bits=10  bin_pt=0  load_pin=off  rst=on  en=off  explicit_period=off  period=1  dbl_ovrd=off  use_behavioral_HDL=off  implementation=Fabric  use_rpm=on  block_type=counter
  Delay : xbsIndex_r4/Delay  en=off  latency=1  dbl_ovrd=off  reg_retiming=off  block_type=delay
  Mux{,1..3} (4 alike) : xbsIndex_r4/Mux  inputs=2  en=off  latency=1  precision=Full  arith_type="Signed  (2's comp)"  n_bits=8  bin_pt=2  quantization=Truncate  overflow=Wrap  dbl_ovrd=off  block_type=mux
  Relational : xbsIndex_r4/Relational  mode=a=b  en=off  latency=1  dbl_ovrd=off  block_type=relational
  Relational1 : xbsIndex_r4/Relational  mode=a=b  en=off  latency=1  dbl_ovrd=off  block_type=relational
  double_delay_bram_fast : monroe_library/double_delay_bram_fast  SystemSampleTime=-1  delay_len=512  bram_latency=2  register_counter=0
  dual_bit_reverse : Subsystem
  unscr_tail : monroe_library/unscr_tail  SystemSampleTime=-1  FFTSize=10  input_bit_width=18  bram_latency=2  reorder_din_latency=0
      link override sync_delay_fast/Constant2: opselect=C  inp2=PCIN>>17  inp1=P  carry=CIN
  pol1_out : Outport
  pol2_out : Outport  Port=2
  pol3_out : Outport  Port=3
  pol4_out : Outport  Port=4
  sync_out : Outport  Port=5
  wires:
  Constant2/1 -> Relational/2
  Constant1/1 -> Relational1/1
  Mux1/1 -> double_delay_bram_fast/1
  Mux/1 -> double_delay_bram_fast/2  "xlsub2_Mux_out1"
  sync/1 -> dual_bit_reverse/1(sync)
  even/1 -> dual_bit_reverse/2(din0)
  odd/1 -> dual_bit_reverse/3(din1)
  dual_bit_reverse/3(dout1) -> Delay/1
  double_delay_bram_fast/1 -> unscr_tail/2
  double_delay_bram_fast/2 -> unscr_tail/3
  Mux3/1 -> unscr_tail/4
  Mux2/1 -> unscr_tail/5
  unscr_tail/1 -> sync_out/1
  unscr_tail/2 -> pol1_out/1
  unscr_tail/3 -> pol2_out/1
  unscr_tail/4 -> pol3_out/1
  unscr_tail/5 -> pol4_out/1
  dual_bit_reverse/2(dout0) -> Mux/3, Mux1/2, Mux2/3, Mux3/2
  dual_bit_reverse/1(sync_out) -> Counter/1, unscr_tail/1
  Relational1/1 -> Mux1/1, Mux2/1
  Relational/1 -> Mux/1, Mux3/1
  Counter/1 -> Relational/1, Relational1/2
  Delay/1 -> Mux/2, Mux1/3, Mux2/2, Mux3/3
